simulink model "flamepropagation"  (R2019b)
settings: Solver=ode45  StartTime=0.0  StopTime=2e4  FixedStep=100  RelTol=1e-3  EnableMultiTasking=on
StartFcn:
  | cput=cputime;
StopFcn:
  | disp('CPU Time Elapsed:');cputime-cput
Description:
  | File Name:  flamepropagation
  | 
  | Purpose:  Illustration of a stiff system
  | 
  | Details:
  | 
  | A model of flame propagation provides an example. This example was derived
  | by Larry Shampine, one of the authors of the MATLAB ODE suite. When you
  | light a match, the ball of flame grows rapidly until it reaches a critical
  | size. Then it remains at that size because the amount of oxygen being
  | consumed by the combustion in the interior of the ball balances the amount
  | available through the surface. The simple model is
  | 
  | ydot = y^2 * ( 1 - y )
  | 
  | This problem is not stiff initially. It only becomes stiff as the solution
  | approaches steady state. This is because the steady-state solution is so
  | "rigid." Any solution near y(t) = 1 increases or decreases rapidly toward
  | that solution. "Rapidly" here is with respect to an unusually long time
  | scale.
  | 
  | You will see that it takes a longer time and uses more timesteps to solve this
  | problem using a non-stiff solver such as ode45 compared to a stiff solver such
  | as ode23s.
settings Model: ExtModeTrigMode=oneshot  ExtModeArmWhenConnect=off  Creator=nicholas  LastModifiedBy=khung
settings DataIOCC: SaveFormat=Array  ReturnWorkspaceOutputs=off
settings OptimizationCC: BlockReduction=off  BooleanDataType=off  ExpressionDepthLimit=2147483647  InitFltsAndDblsToZero=on  LifeSpan=inf
settings DebuggingCC: SaveWithParameterizedLinksMsg=none  UnderspecifiedInitializationDetection=Classic  MergeDetectMultiDrivingBlocksExec=none  SignalResolutionControl=TryResolveAllWithWarning  MultiTaskDSMMsg=warning  MultiTaskCondExecSysMsg=none  ParameterPrecisionLossMsg=none  FcnCallInpInsideContextMsg=warning  StateNameClashWarn=warning  SFUnexpectedBacktrackingDiag=warning  SFNoUnconditionalDefaultTransitionDiag=warning  SFExecutionAtInitializationDiag=none  ArithmeticOperatorsInVariantConditions=warning
settings HardwareCC: ProdBitPerPointer=32  ProdBitPerSizeT=32  ProdBitPerPtrDiffT=32  ProdLargestAtomicFloat=None  ProdIntDivRoundTo=Undefined  ProdEndianess=Unspecified  ProdWordSize=32  ProdHWDeviceType=32-bit Generic  TargetUnknown=on
settings ModelReferenceCC: PropagateSignalLabelsOutOfModel=off
settings SFSimCC: SimUseLocalCustomCode=off  CustomCodeUndefinedFunction=UseInterfaceOnly
settings RTWCC: RTWUseLocalCustomCode=off
settings CodeAppCC: StateflowObjectComments=on
settings GRTTargetCC: TargetFcnLib=ansi_tfl_tmw.mat  TargetLangStandard=C89/C90 (ANSI)  GeneratePreprocessorConditionals=Disable all  CombineOutputUpdateFcns=off  GRTInterface=on
settings ConfigComp: CovMetricSettings=dw  CovHtmlReporting=on  CovSaveCumulativeToWorkspaceVar=on  CovSaveSingleToWorkspaceVar=on  CovExternalEMLEnable=off

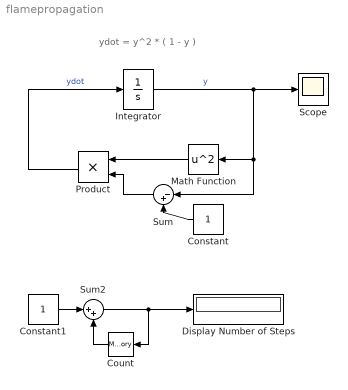
== system flamepropagation ==
  note: ydot = y^2 * ( 1 - y )
  Constant : Constant
  Constant1 : Constant
  Count : Memory
  Display Number of Steps : Display
  Integrator : Integrator  InitialCondition=1e-4
  Math Function : Math  Operator=square  SaturateOnIntegerOverflow=on
  Product : Product  SaturateOnIntegerOverflow=on  RndMeth=Zero  InputSameDT=on  OutDataTypeStr=Inherit: Same as first input
  Scope : Scope
  Sum : Sum  Inputs=|-+  SaturateOnIntegerOverflow=on  InputSameDT=on  OutDataTypeStr=Inherit: Same as first input
  Sum2 : Sum  Inputs=|++  SaturateOnIntegerOverflow=on  InputSameDT=on  OutDataTypeStr=Inherit: Same as first input
  wires:
  Math Function/1 -> Product/1
  Product/1 -> Integrator/1  "ydot"
  Constant/1 -> Sum/2
  Sum/1 -> Product/2
  Integrator/1 -> Math Function/1, Sum/1, Scope/1  "y"
  Constant1/1 -> Sum2/1
  Sum2/1 -> Display Number of Steps/1, Count/1
  Count/1 -> Sum2/2
